simulink model "rst_auto_reg_Prototipo"  (R2015a)
settings: Solver=ode45  SolverMode=SingleTasking  StartTime=0.0  StopTime=50  RelTol=1e-3
values from neighbouring files (symbols this model uses):
  A = den    [cod_teste_RST_4.m]
  B = num    [cod_teste_RST_4.m]
  ep = 0.9    [cod_teste_RST_4.m]
  T = sum(Am)/sum(B)    [cod_teste_RST_4.m]
  Ts = 1    [cod_teste_RST_4.m]
undefined symbols (not defined in the file or in its folder): T_a
libraries: dspinverses x5
settings Model: CovMetricSettings=dwe  CovHtmlReporting=off  covSaveCumulativeToWorkspaceVar=off  CovSaveSingleToWorkspaceVar=off  CovExternalEMLEnable=on  Creator=Carlos Henrique  LastModifiedBy=controle
settings DataIOCC: LimitDataPoints=off  SaveFormat=Dataset
settings DebuggingCC: SFUnexpectedBacktrackingDiag=error  SFNoUnconditionalDefaultTransitionDiag=error
settings HardwareCC: ProdBitPerPointer=64  ProdLargestAtomicFloat=Float  ProdIntDivRoundTo=Zero  ProdEndianess=LittleEndian  ProdHWDeviceType=Specified
settings ModelReferenceCC: PropagateSignalLabelsOutOfModel=on
settings SFSimCC: SimUseLocalCustomCode=on
settings RTWCC: RTWUseLocalCustomCode=on
settings GRTTargetCC: TargetLangStandard=C99 (ISO)  GeneratePreprocessorConditionals=Use local settings

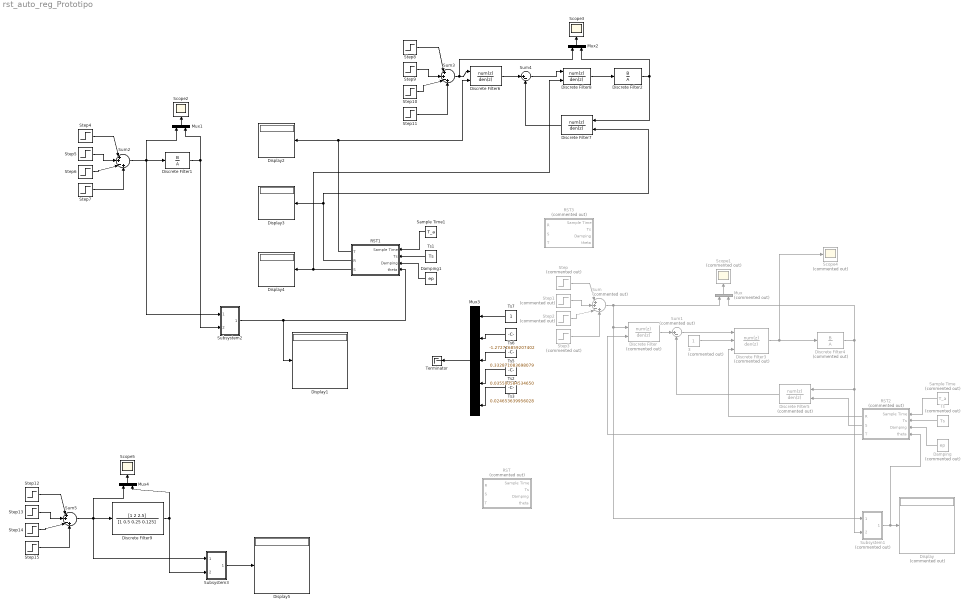
== system rst_auto_reg_Prototipo ==
  3 : Constant  Commented=on
  Damping : Constant  Commented=on  Value=ep
  Damping1 : Constant  Value=ep
  Discrete Filter : DiscreteFilter  Commented=on  NumeratorSource=Input port  Numerator=B  Denominator=1
      settings: InputPortMap=u0,p1
  Discrete Filter1 : DiscreteFilter  Numerator=B  Denominator=A  SampleTime=0.1
  Discrete Filter2 : DiscreteFilter  Numerator=B  Denominator=A  SampleTime=0.1
  Discrete Filter3 : DiscreteFilter  Commented=on  NumeratorSource=Input port  Numerator=T  DenominatorSource=Input port  Denominator=1  SampleTime=0.1  a0EqualsOne=on
      settings: InputPortMap=u0,p1,p3
  Discrete Filter4 : DiscreteFilter  Commented=on  Numerator=B  Denominator=A
  Discrete Filter5 : DiscreteFilter  Commented=on  NumeratorSource=Input port  Denominator=1
      settings: InputPortMap=u0,p1
  Discrete Filter6 : DiscreteFilter  NumeratorSource=Input port  Numerator=13.39  Denominator=1  SampleTime=0.1
      settings: InputPortMap=u0,p1
  Discrete Filter7 : DiscreteFilter  NumeratorSource=Input port  Numerator=[-0.6555 0.1406]  Denominator=1  SampleTime=0.1
      settings: InputPortMap=u0,p1
  Discrete Filter8 : DiscreteFilter  Numerator=1  DenominatorSource=Input port  Denominator=[0.634 -0.2621]  SampleTime=0.1  a0EqualsOne=on
      settings: InputPortMap=u0,p3
  Discrete Filter9 : DiscreteFilter  Numerator=[1 2 2.5]  Denominator=[1 0.5 0.25 0.125]  SampleTime=0.1
  Display : Display  Commented=on
  Display{1..5} (5 alike) : Display
  Mux : Mux  Commented=on  Inputs=2
  Mux1 : Mux  Inputs=2
  Mux2 : Mux  Inputs=2
  Mux3 : Mux  Inputs=5
  Mux4 : Mux  Inputs=2
  RST : Subsystem  Commented=on
  RST1 : Subsystem
  RST2 : Subsystem  Commented=on
  RST3 : Subsystem  Commented=on
  Sample Time : Constant  Commented=on  Value=T_a
  Sample Time1 : Constant  Value=T_a
  Scope1 : Scope  Commented=on
      settings: YMin=-0.73435  YMax=6.60919
  Scope2 : Scope
      settings: YMin=-0.73435  YMax=6.60919
  Scope3 : Scope
      settings: TimeRange=50  YMin=1.132890365448505  YMax=3.006644518272426  SaveName=ScopeData3
  Scope4 : Scope  Commented=on
      settings: YMin=-8.49296  YMax=18.39504  SaveName=ScopeData2
  Scope5 : Scope
      settings: YMin=-0.73435  YMax=6.60919  SaveName=ScopeData4
  Step : Step  Commented=on  Time=0  SampleTime=0
  Step1 : Step  Commented=on  Time=10  After=3  SampleTime=0
  Step10 : Step  Time=20  After=2  SampleTime=0
  Step11 : Step  Time=30  SampleTime=0
  Step12 : Step  Time=0  SampleTime=0
  Step13 : Step  Time=10  After=3  SampleTime=0
  Step14 : Step  Time=20  After=2  SampleTime=0
  Step15 : Step  Time=30  SampleTime=0
  Step2 : Step  Commented=on  Time=20  After=2  SampleTime=0
  Step3 : Step  Commented=on  Time=30  SampleTime=0
  Step4 : Step  Time=0  SampleTime=0
  Step5 : Step  Time=10  After=3  SampleTime=0
  Step6 : Step  Time=20  After=2  SampleTime=0
  Step7 : Step  Time=30  SampleTime=0
  Step8 : Step  Time=0  SampleTime=0
  Step9 : Step  Time=10  After=3  SampleTime=0
  Subsystem1 : Subsystem  Commented=on
  Subsystem2 : Subsystem
  Subsystem3 : Subsystem
  Sum : Sum  Commented=on  Inputs=|++-+
  Sum1 : Sum  Commented=on  Inputs=|+-
  Sum2 : Sum  Inputs=|++-+
  Sum3 : Sum  Inputs=|++-+
  Sum4 : Sum  Inputs=|+-
  Sum5 : Sum  Inputs=|++-+
  Terminator : Terminator
  Ts : Constant  Commented=on  Value=Ts
  Ts1 : Constant  Value=Ts
  Ts2 : Constant  Value=0.035500584534650  SampleTime=0.1
  Ts3 : Constant  Value=0.024653639956028  SampleTime=0.1
  Ts5 : Constant  Value=0.332871083698079  SampleTime=0.1
  Ts6 : Constant  Value=-1.272716859207402  SampleTime=0.1
  Ts7 : Constant  SampleTime=0.1
  wires:
  RST2/2(S) -> Discrete Filter5/2
  Mux/1 -> Scope1/1
  Ts/1 -> RST2/2(Ts)
  Step2/1 -> Sum/3
  Damping/1 -> RST2/3(Damping)
  RST2/1(R) -> Discrete Filter3/3
  Step1/1 -> Sum/2
  Discrete Filter3/1 -> Discrete Filter4/1, Scope4/1
  Sample Time/1 -> RST2/1(Sample Time)
  Sum/1 -> Subsystem1/1(In1), Discrete Filter/1, Mux/1
  Step3/1 -> Sum/4
  3/1 -> Discrete Filter3/2
  Sum1/1 -> Discrete Filter3/1
  Step/1 -> Sum/1
  RST2/3(T) -> Discrete Filter/2
  Discrete Filter/1 -> Sum1/1
  Discrete Filter5/1 -> Sum1/2
  Discrete Filter4/1 -> Subsystem1/2(In2), Discrete Filter5/1, Mux/2
  Sample Time1/1 -> RST1/1(Sample Time)
  Ts1/1 -> RST1/2(Ts)
  Damping1/1 -> RST1/3(Damping)
  Subsystem2/1(Out1) -> Display1/1, RST1/4(theta)
  Step5/1 -> Sum2/2
  Step7/1 -> Sum2/4
  Step6/1 -> Sum2/3
  Step4/1 -> Sum2/1
  Sum2/1 -> Subsystem2/1(In1), Mux1/1, Discrete Filter1/1
  Discrete Filter1/1 -> Subsystem2/2(In2), Mux1/2
  Mux1/1 -> Scope2/1
  RST1/1(T) -> Discrete Filter6/2, Display2/1
  Step8/1 -> Sum3/1
  Step10/1 -> Sum3/3
  Step11/1 -> Sum3/4
  Step9/1 -> Sum3/2
  Sum3/1 -> Mux2/1, Discrete Filter6/1
  Discrete Filter6/1 -> Sum4/1
  Discrete Filter7/1 -> Sum4/2
  Discrete Filter8/1 -> Discrete Filter2/1
  Discrete Filter2/1 -> Discrete Filter7/1, Mux2/2
  Subsystem1/1(Out1) -> RST2/4(theta), Display/1
  Ts7/1 -> Mux3/1
  Ts6/1 -> Mux3/2
  Ts5/1 -> Mux3/3
  Ts2/1 -> Mux3/4
  Ts3/1 -> Mux3/5
  Mux3/1 -> Terminator/1
  RST1/3(S) -> Discrete Filter8/2, Display4/1
  RST1/2(R) -> Discrete Filter7/2, Display3/1
  Sum4/1 -> Discrete Filter8/1
  Mux2/1 -> Scope3/1
  Step13/1 -> Sum5/2
  Step15/1 -> Sum5/4
  Step14/1 -> Sum5/3
  Step12/1 -> Sum5/1
  Sum5/1 -> Discrete Filter9/1, Mux4/1, Subsystem3/1(In1)
  Mux4/1 -> Scope5/1
  Subsystem3/1(Out1) -> Display5/1
  Discrete Filter9/1 -> Subsystem3/2(In2), Mux4/2

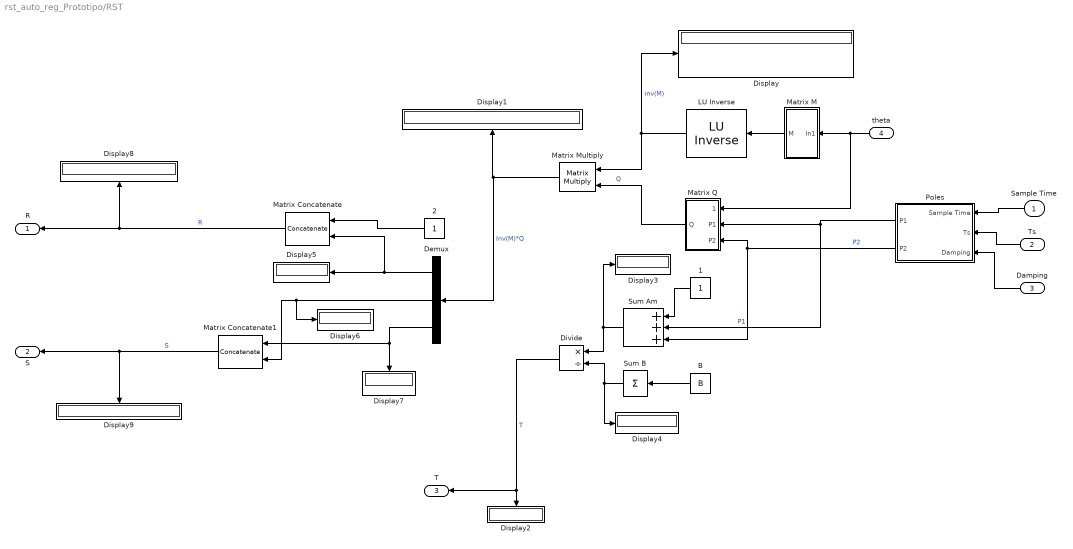
== system rst_auto_reg_Prototipo/RST ==
  Sample Time : Inport
  Ts : Inport  Port=2
  Damping : Inport  Port=3
  theta : Inport  Port=4
  " LU Inverse" : dspinverses/ LU Inverse
  1 : Constant
  2 : Constant
  B : Constant  Value=B
  Demux : Demux  Outputs=3
  Display{,1..9} (10 alike) : Display
  Divide : Product  Inputs=*/
  Matrix Concatenate : Concatenate  Mode=Multidimensional array  ConcatenateDimension=2
  Matrix Concatenate1 : Concatenate  Mode=Multidimensional array  ConcatenateDimension=2
  Matrix M : Subsystem
  Matrix Multiply : Product  Multiplication=Matrix(*)
  Matrix Q : Subsystem
  Poles : Subsystem
  Sum Am : Sum  Inputs=+++
  Sum B : Sum  Inputs=+
  R : Outport
  S : Outport  Port=2
  T : Outport  Port=3
  wires:
  Matrix Multiply/1 -> Demux/1, Display1/1  "Inv(M)*Q"
  Demux/1 -> Matrix Concatenate/2, Display5/1
  Sum B/1 -> Divide/2, Display4/1
  " LU Inverse"/1 -> Matrix Multiply/1, Display/1  "inv(M)"
  Matrix Concatenate/1 -> Display8/1, R/1  "R"
  B/1 -> Sum B/1
  Demux/2 -> Display6/1, Matrix Concatenate1/2
  Sum Am/1 -> Divide/1, Display3/1
  Matrix Concatenate1/1 -> S/1, Display9/1  "S"
  Poles/2(P2) -> Sum Am/3, Matrix Q/3(P2)  "P2"
  Divide/1 -> T/1, Display2/1  "T"
  Ts/1 -> Poles/2(Ts)
  Matrix Q/1(Q) -> Matrix Multiply/2  "Q"
  Damping/1 -> Poles/3(Damping)
  Sample Time/1 -> Poles/1(Sample Time)
  1/1 -> Sum Am/1
  Demux/3 -> Display7/1, Matrix Concatenate1/1
  2/1 -> Matrix Concatenate/1
  theta/1 -> Matrix Q/1(theta), Matrix M/1(In1)
  Matrix M/1(M) -> " LU Inverse"/1
  Poles/1(P1) -> Sum Am/2, Matrix Q/2(P1)  "P1"

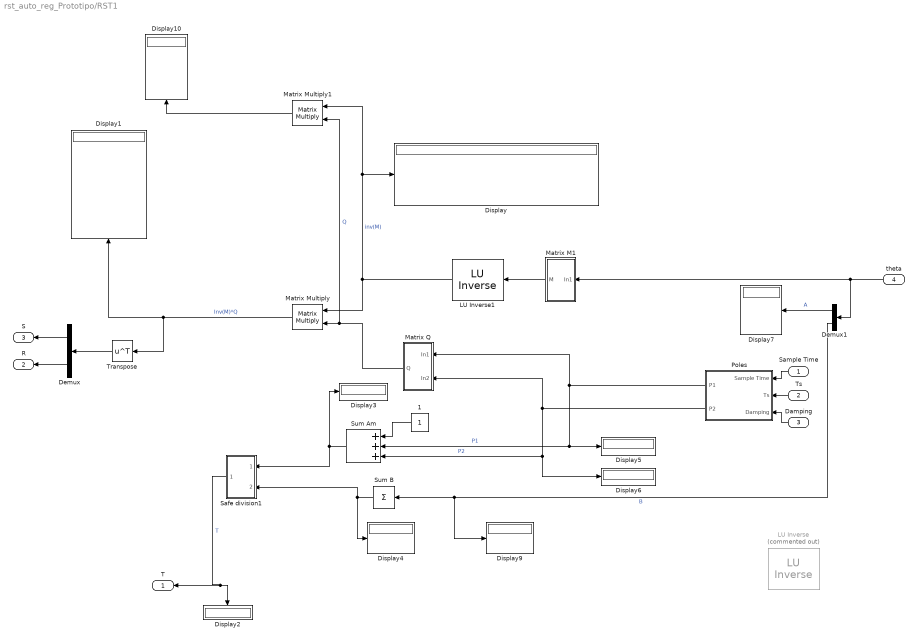
== system rst_auto_reg_Prototipo/RST1 ==
  Sample Time : Inport
  Ts : Inport  Port=2
  Damping : Inport  Port=3
  theta : Inport  Port=4
  " LU Inverse" : dspinverses/ LU Inverse  Commented=on
  " LU Inverse1" : dspinverses/ LU Inverse
  1 : Constant
  Demux : Demux  Outputs=2
  Demux1 : Demux  Outputs=2
  Display{,1..7,9..10} (10 alike) : Display
  Matrix M1 : Subsystem
  Matrix Multiply : Product  Multiplication=Matrix(*)
  Matrix Multiply1 : Product  Multiplication=Matrix(*)
  Matrix Q : Subsystem
  Poles : Subsystem
  Safe division1 : Subsystem
  Sum Am : Sum  Inputs=+++
  Sum B : Sum  Inputs=+
  Transpose : Math  Operator=transpose  SaturateOnIntegerOverflow=on
  T : Outport
  R : Outport  Port=2
  S : Outport  Port=3
  wires:
  Matrix Multiply/1 -> Transpose/1, Display1/1  "Inv(M)*Q"
  Sum B/1 -> Display4/1, Safe division1/2(In2)
  " LU Inverse1"/1 -> Matrix Multiply/1, Matrix Multiply1/1, Display/1  "inv(M)"
  Sum Am/1 -> Safe division1/1(In1), Display3/1
  Safe division1/1(Out1) -> Display2/1, T/1  "T"
  Ts/1 -> Poles/2(Ts)
  Matrix Q/1(Q) -> Matrix Multiply1/2, Matrix Multiply/2  "Q"
  Damping/1 -> Poles/3(Damping)
  Sample Time/1 -> Poles/1(Sample Time)
  1/1 -> Sum Am/1
  theta/1 -> Matrix M1/1(In1), Demux1/1
  Demux1/2 -> Display9/1, Sum B/1  "B"
  Demux1/1 -> Display7/1  "A"
  Poles/1(P1) -> Matrix Q/1(In1), Sum Am/2, Display5/1  "P1"
  Poles/2(P2) -> Display6/1, Sum Am/3, Matrix Q/2(In2)  "P2"
  Matrix M1/1(M) -> " LU Inverse1"/1
  Transpose/1 -> Demux/1
  Demux/1 -> S/1
  Demux/2 -> R/1
  Matrix Multiply1/1 -> Display10/1

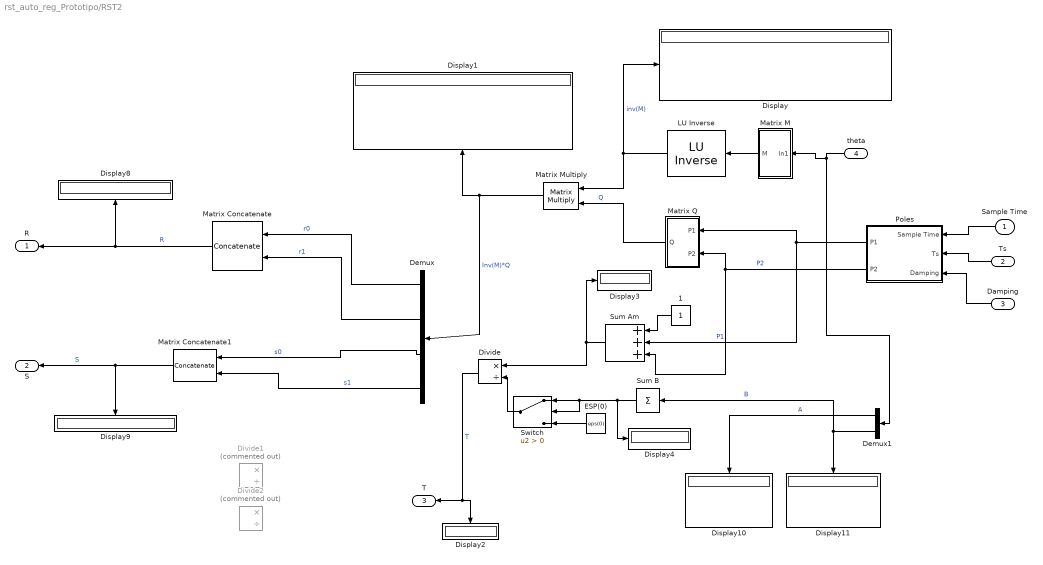
== system rst_auto_reg_Prototipo/RST2 ==
  Sample Time : Inport
  Ts : Inport  Port=2
  Damping : Inport  Port=3
  theta : Inport  Port=4
  " ESP(0)" : Constant  Value=eps(0)
  " LU Inverse" : dspinverses/ LU Inverse
  1 : Constant
  Demux : Demux
  Demux1 : Demux  Outputs=2
  Display{,1..4,8..11} (9 alike) : Display
  Divide : Product  Inputs=*/
  Divide1 : Product  Commented=on  Inputs=*/
  Divide2 : Product  Commented=on  Inputs=*/
  Matrix Concatenate : Concatenate  Mode=Multidimensional array  ConcatenateDimension=2
  Matrix Concatenate1 : Concatenate  Mode=Multidimensional array  ConcatenateDimension=2
  Matrix M : Subsystem
  Matrix Multiply : Product  Multiplication=Matrix(*)
  Matrix Q : Subsystem
  Poles : Subsystem
  Sum Am : Sum  Inputs=+++
  Sum B : Sum  Inputs=+
  Switch : Switch  Criteria=u2 > Threshold
  R : Outport
  S : Outport  Port=2
  T : Outport  Port=3
  wires:
  Demux/4 -> Matrix Concatenate1/2  "s1"
  Demux/3 -> Matrix Concatenate1/1  "s0"
  " ESP(0)"/1 -> Switch/3
  Switch/1 -> Divide/2
  Demux/2 -> Matrix Concatenate/2  "r1"
  Demux/1 -> Matrix Concatenate/1  "r0"
  Demux1/1 -> Display10/1  "A"
  Demux1/2 -> Display11/1, Sum B/1  "B"
  Poles/1(P1) -> Matrix Q/1(P1), Sum Am/2  "P1"
  Matrix M/1(M) -> " LU Inverse"/1
  theta/1 -> Matrix M/1(In1), Demux1/1
  1/1 -> Sum Am/1
  Sample Time/1 -> Poles/1(Sample Time)
  Damping/1 -> Poles/3(Damping)
  Matrix Q/1(Q) -> Matrix Multiply/2  "Q"
  Ts/1 -> Poles/2(Ts)
  Divide/1 -> T/1, Display2/1  "T"
  Poles/2(P2) -> Sum Am/3, Matrix Q/2(P2)  "P2"
  Matrix Concatenate1/1 -> Display9/1, S/1  "S"
  Sum Am/1 -> Display3/1, Divide/1
  Matrix Concatenate/1 -> R/1, Display8/1  "R"
  " LU Inverse"/1 -> Display/1, Matrix Multiply/1  "inv(M)"
  Sum B/1 -> Display4/1, Switch/1, Switch/2
  Matrix Multiply/1 -> Display1/1, Demux/1  "Inv(M)*Q"

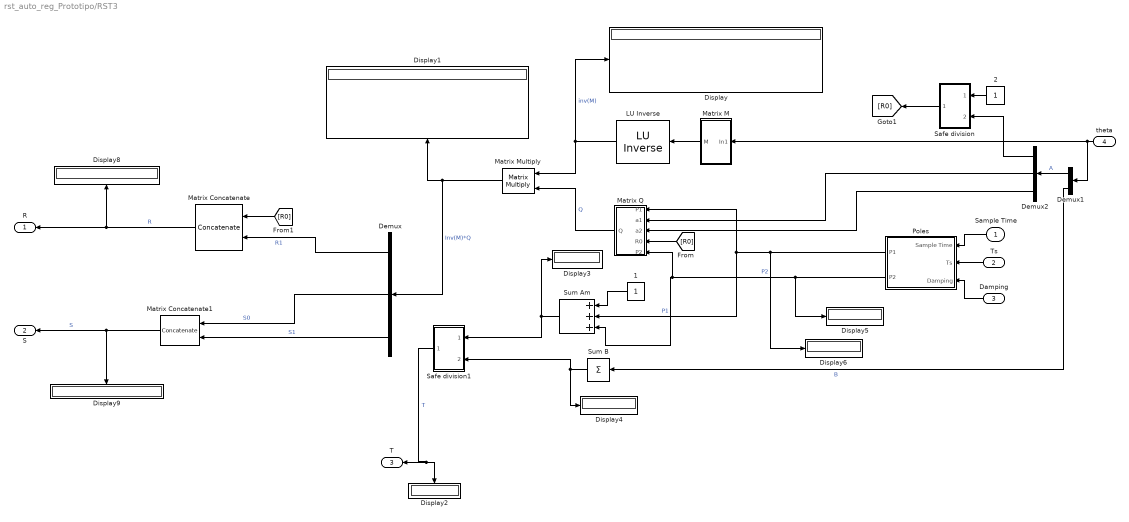
== system rst_auto_reg_Prototipo/RST3 ==
  Sample Time : Inport
  Ts : Inport  Port=2
  Damping : Inport  Port=3
  theta : Inport  Port=4
  " LU Inverse" : dspinverses/ LU Inverse
  1 : Constant
  2 : Constant
  Demux : Demux  Outputs=3
  Demux1 : Demux  Outputs=2
  Demux2 : Demux  Outputs=3
  Display{,1..6,8..9} (9 alike) : Display
  Matrix Concatenate : Concatenate  Mode=Multidimensional array  ConcatenateDimension=2
  Matrix Concatenate1 : Concatenate  Mode=Multidimensional array  ConcatenateDimension=2
  Matrix M : Subsystem
  Matrix Multiply : Product  Multiplication=Matrix(*)
  Matrix Q : Subsystem
  Poles : Subsystem
  Safe division : Subsystem
  Safe division1 : Subsystem
  Sum Am : Sum  Inputs=+++
  Sum B : Sum  Inputs=+
  R : Outport
  S : Outport  Port=2
  T : Outport  Port=3
  wires:
  Demux/1 -> Matrix Concatenate/2  "R1"
  Demux/3 -> Matrix Concatenate1/2  "S1"
  [R0] -> Matrix Concatenate/1
  [R0] -> Matrix Q/4(R0)
  Safe division/1(Out1) -> [R0]
  Demux/2 -> Matrix Concatenate1/1  "S0"
  Demux2/3 -> Matrix Q/3(a2)
  Demux2/2 -> Matrix Q/2(a1)
  2/1 -> Safe division/1(In1)
  Demux2/1 -> Safe division/2(In2)
  Demux1/1 -> Demux2/1  "A"
  Demux1/2 -> Sum B/1  "B"
  Poles/1(P1) -> Sum Am/2, Matrix Q/1(P1), Display6/1  "P1"
  Matrix M/1(M) -> " LU Inverse"/1
  theta/1 -> Demux1/1, Matrix M/1(In1)
  1/1 -> Sum Am/1
  Sample Time/1 -> Poles/1(Sample Time)
  Damping/1 -> Poles/3(Damping)
  Matrix Q/1(Q) -> Matrix Multiply/2  "Q"
  Ts/1 -> Poles/2(Ts)
  Safe division1/1(Out1) -> T/1, Display2/1  "T"
  Poles/2(P2) -> Sum Am/3, Matrix Q/5(P2), Display5/1  "P2"
  Matrix Concatenate1/1 -> S/1, Display9/1  "S"
  Sum Am/1 -> Display3/1, Safe division1/1(In1)
  Matrix Concatenate/1 -> R/1, Display8/1  "R"
  " LU Inverse"/1 -> Display/1, Matrix Multiply/1  "inv(M)"
  Sum B/1 -> Safe division1/2(In2), Display4/1
  Matrix Multiply/1 -> Display1/1, Demux/1  "Inv(M)*Q"

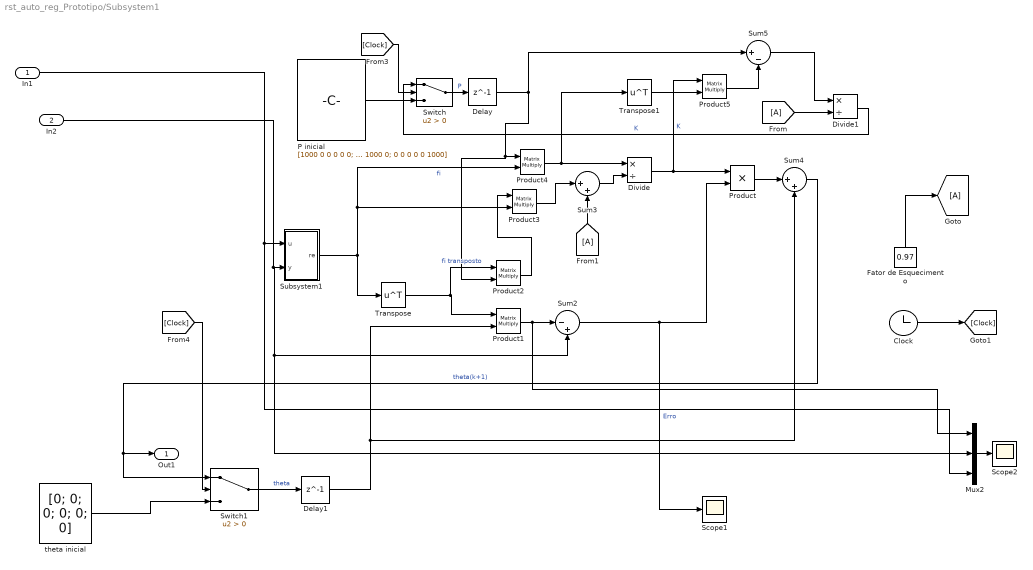
== system rst_auto_reg_Prototipo/Subsystem1 ==
  In1 : Inport
  In2 : Inport  Port=2
  Clock : Clock
  Delay : Delay  DelayLength=1  InitialCondition=0  SampleTime=0.1
  Delay1 : Delay  DelayLength=1  InitialCondition=0  SampleTime=0.1
  Divide : Product  Inputs=*/
  Divide1 : Product  Inputs=*/
  "Fator de Esquecimento " : Constant  Value=0.97
  Mux2 : Mux  Inputs=3
  P inicial : Constant  Value=[1000 0 0 0 0 0; 0 1000 0 0 0 0; 0 0 1000 0 0 0; 0 0 0 1000 0 0; 0 0 0 0 1000 0; 0 0 0 0 0 1000]
  Product : Product
  Product{1..5} (5 alike) : Product  Multiplication=Matrix(*)
  Scope1 : Scope
      settings: YMin=-0.1368  YMax=1.23123
  Scope2 : Scope
      settings: YMin=-0.50752  YMax=4.51143
  Subsystem1 : Subsystem
  Sum2 : Sum  Inputs=|-+
  Sum3 : Sum  Inputs=|++
  Sum4 : Sum  Inputs=|++
  Sum5 : Sum  Inputs=|+-
  Switch : Switch  Criteria=u2 > Threshold
  Switch1 : Switch  Criteria=u2 > Threshold
  Transpose : Math  Operator=transpose  SaturateOnIntegerOverflow=on
  Transpose1 : Math  Operator=transpose  SaturateOnIntegerOverflow=on
  "theta inicial " : Constant  Value=[0; 0; 0; 0; 0; 0]
  Out1 : Outport
  wires:
  Subsystem1/1(re) -> Transpose/1, Product4/2, Product3/2  "fi"
  Product/1 -> Sum4/1
  In2/1 -> Mux2/2, Sum2/2, Subsystem1/2(y)
  "Fator de Esquecimento "/1 -> [A]
  Transpose/1 -> Product2/1, Product1/1  "fi transposto"
  Sum3/1 -> Divide/2
  Product3/1 -> Sum3/1
  Switch/1 -> Delay/1  "P"
  Product4/1 -> Transpose1/1, Divide/1
  Delay/1 -> Product2/2, Product4/1, Sum5/1
  Divide/1 -> Product5/1, Product/1  "K"
  Transpose1/1 -> Product5/2
  Sum5/1 -> Divide1/1
  Sum2/1 -> Scope1/1, Product/2  "Erro"
  Delay1/1 -> Sum4/2, Product1/2
  Divide1/1 -> Switch/1  "K"
  "theta inicial "/1 -> Switch1/3
  [A] -> Divide1/2
  Product2/1 -> Product3/1
  Clock/1 -> [Clock]
  Product1/1 -> Mux2/1, Sum2/1
  Product5/1 -> Sum5/2
  P inicial/1 -> Switch/3
  Sum4/1 -> Out1/1, Switch1/1  "theta(k+1)"
  [A] -> Sum3/2
  In1/1 -> Mux2/3, Subsystem1/1(u)
  [Clock] -> Switch/2
  Switch1/1 -> Delay1/1  "theta"
  Mux2/1 -> Scope2/1
  [Clock] -> Switch1/2

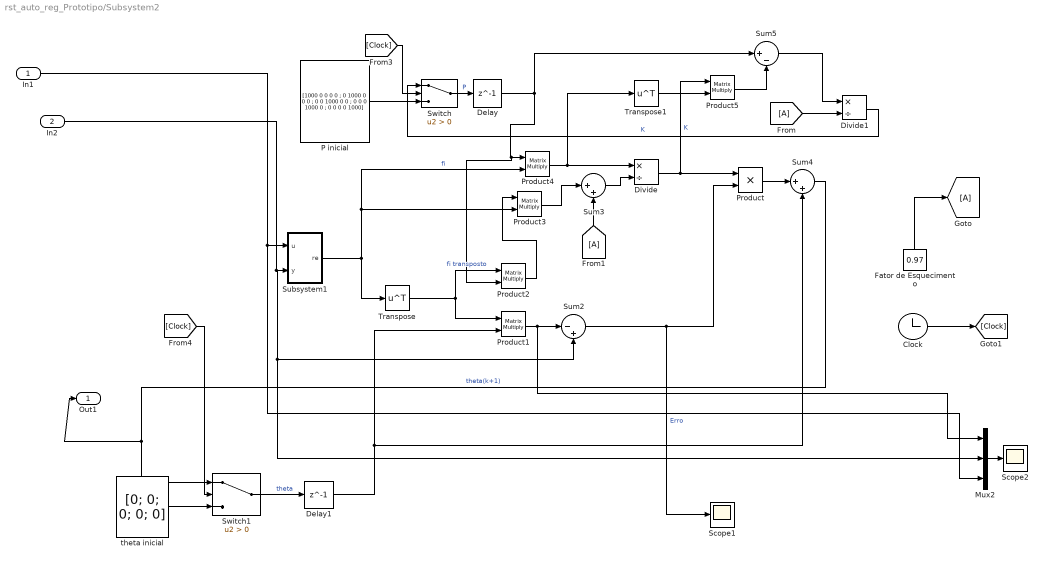
== system rst_auto_reg_Prototipo/Subsystem2 ==
  In1 : Inport
  In2 : Inport  Port=2
  Clock : Clock
  Delay : Delay  DelayLength=1  InitialCondition=0  SampleTime=0.1
  Delay1 : Delay  DelayLength=1  InitialCondition=0  SampleTime=0.1
  Divide : Product  Inputs=*/
  Divide1 : Product  Inputs=*/
  "Fator de Esquecimento " : Constant  Value=0.97
  Mux2 : Mux  Inputs=3
  P inicial : Constant  Value=[1000 0 0 0 0 ; 0 1000 0 0 0 ; 0 0 1000 0 0 ; 0 0 0 1000 0 ; 0 0 0 0 1000]  SampleTime=0.1
  Product : Product
  Product{1..5} (5 alike) : Product  Multiplication=Matrix(*)
  Scope1 : Scope
      settings: YMin=-0.1368  YMax=1.23123
  Scope2 : Scope
      settings: YMin=-0.50752  YMax=4.51143
  Subsystem1 : Subsystem
  Sum2 : Sum  Inputs=|-+
  Sum3 : Sum  Inputs=|++
  Sum4 : Sum  Inputs=|++
  Sum5 : Sum  Inputs=|+-
  Switch : Switch  Criteria=u2 > Threshold
  Switch1 : Switch  Criteria=u2 > Threshold
  Transpose : Math  Operator=transpose  SaturateOnIntegerOverflow=on
  Transpose1 : Math  Operator=transpose  SaturateOnIntegerOverflow=on
  "theta inicial " : Constant  Value=[0; 0; 0; 0; 0]  SampleTime=0.1
  Out1 : Outport
  wires:
  Subsystem1/1(re) -> Transpose/1, Product4/2, Product3/2  "fi"
  Product/1 -> Sum4/1
  In2/1 -> Mux2/2, Sum2/2, Subsystem1/2(y)
  "Fator de Esquecimento "/1 -> [A]
  Transpose/1 -> Product2/1, Product1/1  "fi transposto"
  Sum3/1 -> Divide/2
  Product3/1 -> Sum3/1
  Switch/1 -> Delay/1  "P"
  Product4/1 -> Transpose1/1, Divide/1
  Delay/1 -> Product2/2, Product4/1, Sum5/1
  Divide/1 -> Product5/1, Product/1  "K"
  Transpose1/1 -> Product5/2
  Sum5/1 -> Divide1/1
  Sum2/1 -> Scope1/1, Product/2  "Erro"
  Delay1/1 -> Sum4/2, Product1/2
  Divide1/1 -> Switch/1  "K"
  "theta inicial "/1 -> Switch1/3
  [A] -> Divide1/2
  Product2/1 -> Product3/1
  Clock/1 -> [Clock]
  Product1/1 -> Mux2/1, Sum2/1
  Product5/1 -> Sum5/2
  P inicial/1 -> Switch/3
  Sum4/1 -> Out1/1, Switch1/1  "theta(k+1)"
  [A] -> Sum3/2
  In1/1 -> Mux2/3, Subsystem1/1(u)
  [Clock] -> Switch/2
  Switch1/1 -> Delay1/1  "theta"
  Mux2/1 -> Scope2/1
  [Clock] -> Switch1/2

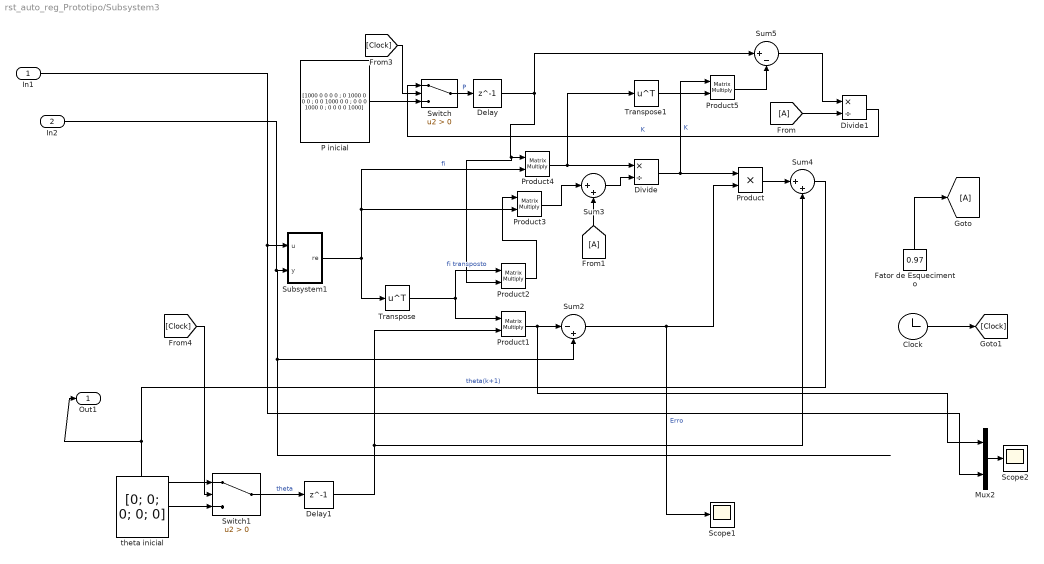
== system rst_auto_reg_Prototipo/Subsystem3 ==
  In1 : Inport
  In2 : Inport  Port=2
  Clock : Clock
  Delay : Delay  DelayLength=1  InitialCondition=0  SampleTime=0.1
  Delay1 : Delay  DelayLength=1  InitialCondition=0  SampleTime=0.1
  Divide : Product  Inputs=*/
  Divide1 : Product  Inputs=*/
  "Fator de Esquecimento " : Constant  Value=0.97
  Mux2 : Mux  Inputs=2
  P inicial : Constant  Value=[1000 0 0 0 0 ; 0 1000 0 0 0 ; 0 0 1000 0 0 ; 0 0 0 1000 0 ; 0 0 0 0 1000]  SampleTime=0.1
  Product : Product
  Product{1..5} (5 alike) : Product  Multiplication=Matrix(*)
  Scope1 : Scope
      settings: YMin=-0.1368  YMax=1.23123
  Scope2 : Scope
      settings: TimeRange=20  YMin=0.1724517906336078  YMax=1.772451790633608
  Subsystem1 : Subsystem
  Sum2 : Sum  Inputs=|-+
  Sum3 : Sum  Inputs=|++
  Sum4 : Sum  Inputs=|++
  Sum5 : Sum  Inputs=|+-
  Switch : Switch  Criteria=u2 > Threshold
  Switch1 : Switch  Criteria=u2 > Threshold
  Transpose : Math  Operator=transpose  SaturateOnIntegerOverflow=on
  Transpose1 : Math  Operator=transpose  SaturateOnIntegerOverflow=on
  "theta inicial " : Constant  Value=[0; 0; 0; 0; 0]  SampleTime=0.1
  Out1 : Outport
  wires:
  Subsystem1/1(re) -> Transpose/1, Product4/2, Product3/2  "fi"
  Product/1 -> Sum4/1
  In2/1 -> Sum2/2, Subsystem1/2(y)
  "Fator de Esquecimento "/1 -> [A]
  Transpose/1 -> Product2/1, Product1/1  "fi transposto"
  Sum3/1 -> Divide/2
  Product3/1 -> Sum3/1
  Switch/1 -> Delay/1  "P"
  Product4/1 -> Transpose1/1, Divide/1
  Delay/1 -> Product2/2, Product4/1, Sum5/1
  Divide/1 -> Product5/1, Product/1  "K"
  Transpose1/1 -> Product5/2
  Sum5/1 -> Divide1/1
  Sum2/1 -> Scope1/1, Product/2  "Erro"
  Delay1/1 -> Sum4/2, Product1/2
  Divide1/1 -> Switch/1  "K"
  "theta inicial "/1 -> Switch1/3
  [A] -> Divide1/2
  Product2/1 -> Product3/1
  Clock/1 -> [Clock]
  Product1/1 -> Mux2/1, Sum2/1
  Product5/1 -> Sum5/2
  P inicial/1 -> Switch/3
  Sum4/1 -> Out1/1, Switch1/1  "theta(k+1)"
  [A] -> Sum3/2
  In1/1 -> Mux2/2, Subsystem1/1(u)
  [Clock] -> Switch/2
  Switch1/1 -> Delay1/1  "theta"
  Mux2/1 -> Scope2/1
  [Clock] -> Switch1/2

== system rst_auto_reg_Prototipo/RST/Matrix M ==
  In1 : Inport
  " " : Constant  Value=0
  1 : Constant
  Demux : Demux  Outputs=6
  Display : Display
  Matrix Concatenate{,1..5} (6 alike) : Concatenate  Mode=Multidimensional array  ConcatenateDimension=2
  Matrix Concatenate6 : Concatenate  Mode=Multidimensional array
  Matrix Concatenate7 : Concatenate  Mode=Multidimensional array
  Terminator : Terminator
  Terminator1 : Terminator
  M : Outport
  wires:
  Demux/6 -> Matrix Concatenate4/2, Matrix Concatenate3/2  "b3"
  Demux/4 -> Terminator/1
  Demux/3 -> Matrix Concatenate4/1  "a3"
  In1/1 -> Demux/1
  Demux/5 -> Matrix Concatenate2/2, Matrix Concatenate1/2  "b2"
  Demux/2 -> Matrix Concatenate2/1  "a2"
  " "/1 -> Matrix Concatenate/2, Matrix Concatenate5/2
  Demux/1 -> Terminator1/1  "a1"
  Matrix Concatenate4/1 -> Matrix Concatenate5/1
  1/1 -> Matrix Concatenate/1
  Matrix Concatenate5/1 -> Matrix Concatenate7/2
  Matrix Concatenate2/1 -> Matrix Concatenate3/1
  Matrix Concatenate/1 -> Matrix Concatenate1/1
  Matrix Concatenate6/1 -> Matrix Concatenate7/1
  Matrix Concatenate3/1 -> Matrix Concatenate6/2
  Matrix Concatenate7/1 -> M/1, Display/1
  Matrix Concatenate1/1 -> Matrix Concatenate6/1

== system rst_auto_reg_Prototipo/RST/Matrix Q ==
  theta : Inport
  P1 : Inport  Port=2
  P2 : Inport  Port=3
  0 : Constant  Value=0
  Demux : Demux  Outputs=6
  Display : Display
  Matrix Concatenate : Concatenate  Mode=Multidimensional array
  Matrix Concatenate1 : Concatenate  Mode=Multidimensional array
  Subtract : Sum  Inputs=+-
  Subtract1 : Sum  Inputs=+-
  Terminator{,1..3} (4 alike) : Terminator
  Q : Outport
  wires:
  Subtract1/1 -> Matrix Concatenate/2
  Matrix Concatenate/1 -> Matrix Concatenate1/1
  Subtract/1 -> Matrix Concatenate/1
  Matrix Concatenate1/1 -> Q/1, Display/1
  P1/1 -> Subtract/1
  0/1 -> Matrix Concatenate1/2
  P2/1 -> Subtract1/1
  theta/1 -> Demux/1
  Demux/6 -> Terminator1/1  "b3"
  Demux/5 -> Terminator/1  "b2"
  Demux/4 -> Terminator2/1
  Demux/1 -> Terminator3/1  "a1"
  Demux/2 -> Subtract/2  "a2"
  Demux/3 -> Subtract1/2  "a3"

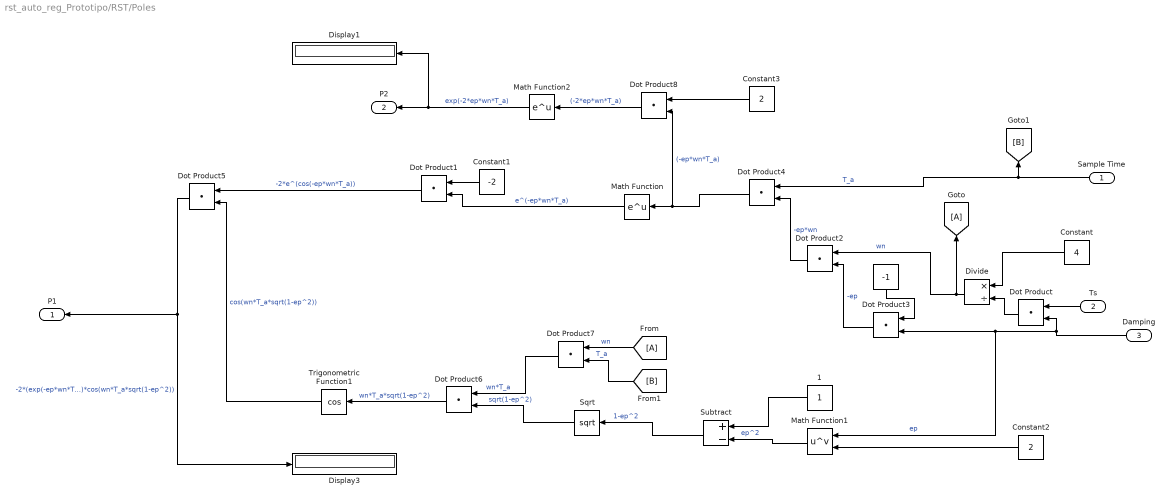
== system rst_auto_reg_Prototipo/RST/Poles ==
  Sample Time : Inport
  Ts : Inport  Port=2
  Damping : Inport  Port=3
  " " : Constant  Value=-1
  1 : Constant
  Constant : Constant  Value=4
  Constant1 : Constant  Value=-2
  Constant2 : Constant  Value=2
  Constant3 : Constant  Value=2
  Display1 : Display
  Display3 : Display
  Divide : Product  Inputs=*/
  Dot Product{,1..8} (9 alike) : DotProduct  InputSameDT=on  OutDataTypeStr=Inherit: Inherit via internal rule
  Math Function : Math  SaturateOnIntegerOverflow=on
  Math Function1 : Math  Operator=pow  SaturateOnIntegerOverflow=on
  Math Function2 : Math  SaturateOnIntegerOverflow=on
  Sqrt : Sqrt  SaturateOnIntegerOverflow=on
  Subtract : Sum  Inputs=+-
  Trigonometric Function1 : Trigonometry  Operator=cos
  P1 : Outport
  P2 : Outport  Port=2
  wires:
  Math Function/1 -> Dot Product1/2  "e^(-ep*wn*T_a)"
  Divide/1 -> [A], Dot Product2/1  "wn"
  [A] -> Dot Product7/1  "wn"
  " "/1 -> Dot Product3/1
  Dot Product5/1 -> P1/1, Display3/1  "-2*(exp(-ep*wn*T_a))*cos(wn*T_a*sqrt(1-ep^2))"
  Trigonometric Function1/1 -> Dot Product5/2  "cos(wn*T_a*sqrt(1-ep^2))"
  Ts/1 -> Dot Product/1
  Dot Product/1 -> Divide/2
  Dot Product3/1 -> Dot Product2/2  "-ep"
  Damping/1 -> Math Function1/1, Dot Product3/2, Dot Product/2  "ep"
  Constant/1 -> Divide/1
  Dot Product7/1 -> Dot Product6/1  "wn*T_a"
  Sample Time/1 -> Dot Product4/1, [B]  "T_a"
  Math Function1/1 -> Subtract/2  "ep^2"
  Dot Product1/1 -> Dot Product5/1  "-2*e^(cos(-ep*wn*T_a))"
  Constant2/1 -> Math Function1/2
  1/1 -> Subtract/1
  Constant1/1 -> Dot Product1/1
  Dot Product2/1 -> Dot Product4/2  "-ep*wn"
  [B] -> Dot Product7/2  "T_a"
  Dot Product6/1 -> Trigonometric Function1/1  "wn*T_a*sqrt(1-ep^2)"
  Dot Product4/1 -> Dot Product8/2, Math Function/1  "(-ep*wn*T_a)"
  Sqrt/1 -> Dot Product6/2  "sqrt(1-ep^2)"
  Subtract/1 -> Sqrt/1  "1-ep^2"
  Constant3/1 -> Dot Product8/1
  Dot Product8/1 -> Math Function2/1  "(-2*ep*wn*T_a)"
  Math Function2/1 -> Display1/1, P2/1  "exp(-2*ep*wn*T_a)"

== system rst_auto_reg_Prototipo/RST1/Matrix M1 ==
  In1 : Inport
  " " : Constant  Value=0
  Demux : Demux  Outputs=5
  Display : Display
  Matrix Concatenate{1..4} (4 alike) : Concatenate  NumInputs=4  Mode=Multidimensional array  ConcatenateDimension=2
  Matrix Concatenate6 : Concatenate  NumInputs=4  Mode=Multidimensional array
  M : Outport
  wires:
  Matrix Concatenate1/1 -> Matrix Concatenate6/1
  Demux/1 -> Matrix Concatenate2/2, Matrix Concatenate1/1  "a0"
  Matrix Concatenate6/1 -> M/1, Display/1
  In1/1 -> Demux/1
  Matrix Concatenate3/1 -> Matrix Concatenate6/3
  Matrix Concatenate4/1 -> Matrix Concatenate6/4
  Matrix Concatenate2/1 -> Matrix Concatenate6/2
  " "/1 -> Matrix Concatenate4/3, Matrix Concatenate4/1, Matrix Concatenate2/4, Matrix Concatenate1/4, Matrix Concatenate1/2, Matrix Concatenate1/3
  Demux/2 -> Matrix Concatenate3/2, Matrix Concatenate2/1  "a1"
  Demux/3 -> Matrix Concatenate4/2, Matrix Concatenate3/1  "a2"
  Demux/4 -> Matrix Concatenate3/4  "b1"
  Demux/5 -> Matrix Concatenate4/4, Matrix Concatenate2/3, Matrix Concatenate3/3  "b2"

== system rst_auto_reg_Prototipo/RST1/Matrix Q ==
  In1 : Inport
  In2 : Inport  Port=2
  0 : Constant  Value=0
  1 : Constant
  Display : Display
  Matrix Concatenate : Concatenate  NumInputs=4  Mode=Multidimensional array
  Q : Outport
  wires:
  Matrix Concatenate/1 -> Q/1, Display/1
  0/1 -> Matrix Concatenate/4
  1/1 -> Matrix Concatenate/1
  In1/1 -> Matrix Concatenate/2
  In2/1 -> Matrix Concatenate/3

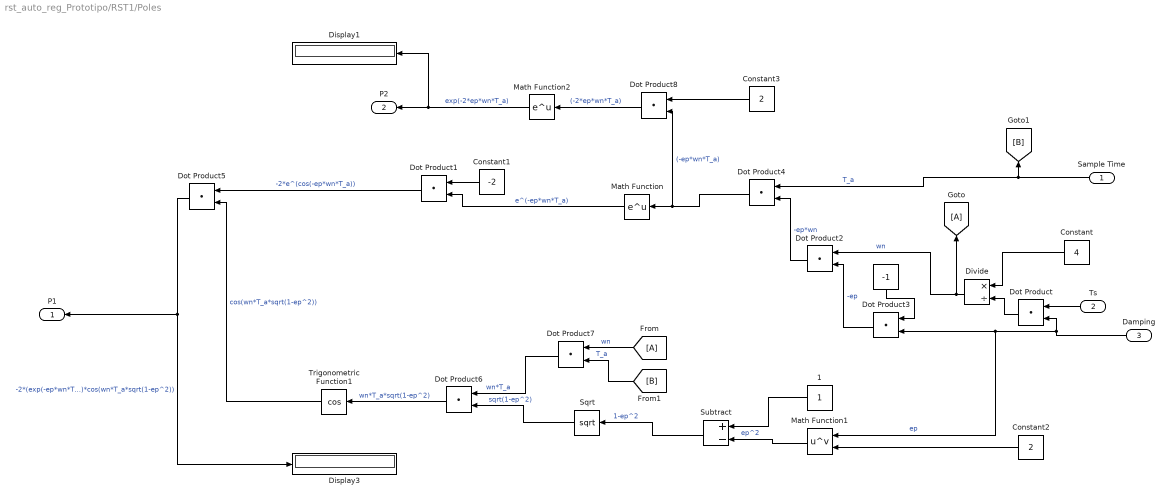
== system rst_auto_reg_Prototipo/RST1/Poles ==
  Sample Time : Inport
  Ts : Inport  Port=2
  Damping : Inport  Port=3
  " " : Constant  Value=-1
  1 : Constant
  Constant : Constant  Value=4
  Constant1 : Constant  Value=-2
  Constant2 : Constant  Value=2
  Constant3 : Constant  Value=2
  Display1 : Display
  Display3 : Display
  Divide : Product  Inputs=*/
  Dot Product{,1..8} (9 alike) : DotProduct  InputSameDT=on  OutDataTypeStr=Inherit: Inherit via internal rule
  Math Function : Math  SaturateOnIntegerOverflow=on
  Math Function1 : Math  Operator=pow  SaturateOnIntegerOverflow=on
  Math Function2 : Math  SaturateOnIntegerOverflow=on
  Sqrt : Sqrt  SaturateOnIntegerOverflow=on
  Subtract : Sum  Inputs=+-
  Trigonometric Function1 : Trigonometry  Operator=cos
  P1 : Outport
  P2 : Outport  Port=2
  wires:
  Math Function/1 -> Dot Product1/2  "e^(-ep*wn*T_a)"
  Divide/1 -> [A], Dot Product2/1  "wn"
  [A] -> Dot Product7/1  "wn"
  " "/1 -> Dot Product3/1
  Dot Product5/1 -> P1/1, Display3/1  "-2*(exp(-ep*wn*T_a))*cos(wn*T_a*sqrt(1-ep^2))"
  Trigonometric Function1/1 -> Dot Product5/2  "cos(wn*T_a*sqrt(1-ep^2))"
  Ts/1 -> Dot Product/1
  Dot Product/1 -> Divide/2
  Dot Product3/1 -> Dot Product2/2  "-ep"
  Damping/1 -> Math Function1/1, Dot Product3/2, Dot Product/2  "ep"
  Constant/1 -> Divide/1
  Dot Product7/1 -> Dot Product6/1  "wn*T_a"
  Sample Time/1 -> Dot Product4/1, [B]  "T_a"
  Math Function1/1 -> Subtract/2  "ep^2"
  Dot Product1/1 -> Dot Product5/1  "-2*e^(cos(-ep*wn*T_a))"
  Constant2/1 -> Math Function1/2
  1/1 -> Subtract/1
  Constant1/1 -> Dot Product1/1
  Dot Product2/1 -> Dot Product4/2  "-ep*wn"
  [B] -> Dot Product7/2  "T_a"
  Dot Product6/1 -> Trigonometric Function1/1  "wn*T_a*sqrt(1-ep^2)"
  Dot Product4/1 -> Dot Product8/2, Math Function/1  "(-ep*wn*T_a)"
  Sqrt/1 -> Dot Product6/2  "sqrt(1-ep^2)"
  Subtract/1 -> Sqrt/1  "1-ep^2"
  Constant3/1 -> Dot Product8/1
  Dot Product8/1 -> Math Function2/1  "(-2*ep*wn*T_a)"
  Math Function2/1 -> Display1/1, P2/1  "exp(-2*ep*wn*T_a)"

== system rst_auto_reg_Prototipo/RST1/Safe division1 ==
  In1 : Inport
  In2 : Inport  Port=2
  " ESP(0)1" : Constant  Value=eps(0)
  Divide3 : Product  Inputs=*/
  Switch1 : Switch  Criteria=u2 > Threshold
  Out1 : Outport
  wires:
  Divide3/1 -> Out1/1
  In1/1 -> Divide3/1
  In2/1 -> Switch1/2, Switch1/1
  " ESP(0)1"/1 -> Switch1/3
  Switch1/1 -> Divide3/2

== system rst_auto_reg_Prototipo/RST2/Matrix M ==
  In1 : Inport
  " " : Constant  Value=0
  Demux : Demux  Outputs=6
  Display : Display
  Matrix Concatenate{,1..3} (4 alike) : Concatenate  NumInputs=4  Mode=Multidimensional array  ConcatenateDimension=2
  Matrix Concatenate6 : Concatenate  NumInputs=4  Mode=Multidimensional array
  M : Outport
  wires:
  Matrix Concatenate3/1 -> Matrix Concatenate6/4
  Matrix Concatenate1/1 -> Matrix Concatenate6/3
  Matrix Concatenate2/1 -> Matrix Concatenate6/2
  Matrix Concatenate/1 -> Matrix Concatenate6/1
  Matrix Concatenate6/1 -> Display/1, M/1
  Demux/6 -> Matrix Concatenate1/3, Matrix Concatenate3/4  "b2"
  Demux/5 -> Matrix Concatenate1/4, Matrix Concatenate2/3  "b1"
  Demux/3 -> Matrix Concatenate1/1, Matrix Concatenate3/2  "a2"
  Demux/2 -> Matrix Concatenate1/2, Matrix Concatenate2/1  "a1"
  Demux/4 -> Matrix Concatenate2/4, Matrix Concatenate/3  "b0"
  " "/1 -> Matrix Concatenate/2, Matrix Concatenate/4, Matrix Concatenate3/1, Matrix Concatenate3/3
  Demux/1 -> Matrix Concatenate2/2, Matrix Concatenate/1  "a0"
  In1/1 -> Demux/1

== system rst_auto_reg_Prototipo/RST2/Matrix Q ==
  P1 : Inport
  P2 : Inport  Port=2
  0 : Constant  Value=0
  1 : Constant
  Display : Display
  Matrix Concatenate : Concatenate  NumInputs=4  Mode=Multidimensional array
  Q : Outport
  wires:
  0/1 -> Matrix Concatenate/4
  P2/1 -> Matrix Concatenate/3
  P1/1 -> Matrix Concatenate/2
  1/1 -> Matrix Concatenate/1
  Matrix Concatenate/1 -> Display/1, Q/1

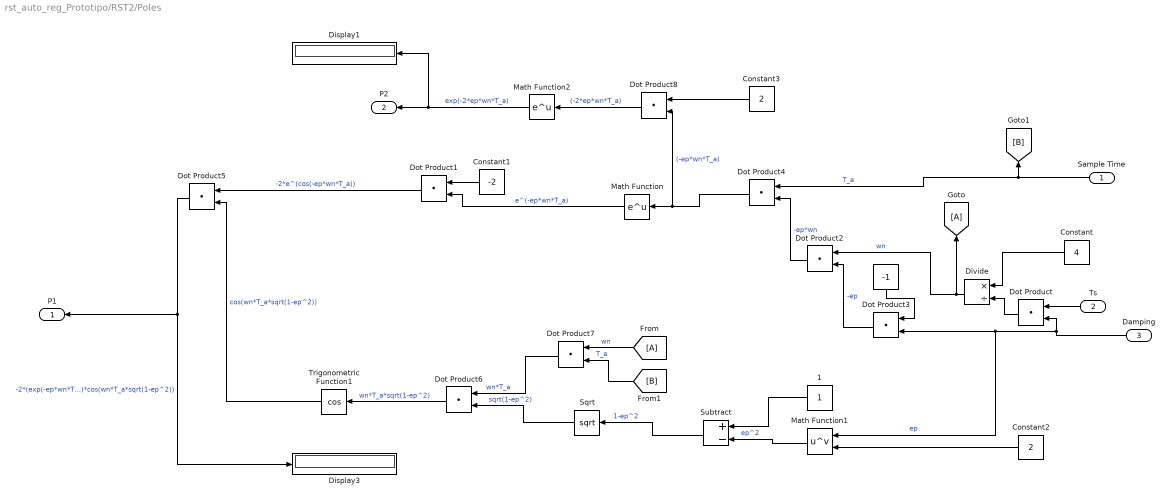
== system rst_auto_reg_Prototipo/RST2/Poles ==
  Sample Time : Inport
  Ts : Inport  Port=2
  Damping : Inport  Port=3
  " " : Constant  Value=-1
  1 : Constant
  Constant : Constant  Value=4
  Constant1 : Constant  Value=-2
  Constant2 : Constant  Value=2
  Constant3 : Constant  Value=2
  Display1 : Display
  Display3 : Display
  Divide : Product  Inputs=*/
  Dot Product{,1..8} (9 alike) : DotProduct  InputSameDT=on  OutDataTypeStr=Inherit: Inherit via internal rule
  Math Function : Math  SaturateOnIntegerOverflow=on
  Math Function1 : Math  Operator=pow  SaturateOnIntegerOverflow=on
  Math Function2 : Math  SaturateOnIntegerOverflow=on
  Sqrt : Sqrt  SaturateOnIntegerOverflow=on
  Subtract : Sum  Inputs=+-
  Trigonometric Function1 : Trigonometry  Operator=cos
  P1 : Outport
  P2 : Outport  Port=2
  wires:
  Math Function2/1 -> P2/1, Display1/1  "exp(-2*ep*wn*T_a)"
  Dot Product8/1 -> Math Function2/1  "(-2*ep*wn*T_a)"
  Constant3/1 -> Dot Product8/1
  Subtract/1 -> Sqrt/1  "1-ep^2"
  Sqrt/1 -> Dot Product6/2  "sqrt(1-ep^2)"
  Dot Product4/1 -> Math Function/1, Dot Product8/2  "(-ep*wn*T_a)"
  Dot Product6/1 -> Trigonometric Function1/1  "wn*T_a*sqrt(1-ep^2)"
  [B] -> Dot Product7/2  "T_a"
  Dot Product2/1 -> Dot Product4/2  "-ep*wn"
  Constant1/1 -> Dot Product1/1
  1/1 -> Subtract/1
  Constant2/1 -> Math Function1/2
  Dot Product1/1 -> Dot Product5/1  "-2*e^(cos(-ep*wn*T_a))"
  Math Function1/1 -> Subtract/2  "ep^2"
  Sample Time/1 -> [B], Dot Product4/1  "T_a"
  Dot Product7/1 -> Dot Product6/1  "wn*T_a"
  Constant/1 -> Divide/1
  Damping/1 -> Dot Product/2, Dot Product3/2, Math Function1/1  "ep"
  Dot Product3/1 -> Dot Product2/2  "-ep"
  Dot Product/1 -> Divide/2
  Ts/1 -> Dot Product/1
  Trigonometric Function1/1 -> Dot Product5/2  "cos(wn*T_a*sqrt(1-ep^2))"
  Dot Product5/1 -> Display3/1, P1/1  "-2*(exp(-ep*wn*T_a))*cos(wn*T_a*sqrt(1-ep^2))"
  " "/1 -> Dot Product3/1
  [A] -> Dot Product7/1  "wn"
  Divide/1 -> Dot Product2/1, [A]  "wn"
  Math Function/1 -> Dot Product1/2  "e^(-ep*wn*T_a)"

== system rst_auto_reg_Prototipo/RST3/Matrix M ==
  In1 : Inport
  " " : Constant  Value=0
  Demux : Demux  Outputs=5
  Display : Display
  Matrix Concatenate1 : Concatenate  NumInputs=3  Mode=Multidimensional array  ConcatenateDimension=2
  Matrix Concatenate2 : Concatenate  NumInputs=3  Mode=Multidimensional array  ConcatenateDimension=2
  Matrix Concatenate3 : Concatenate  NumInputs=3  Mode=Multidimensional array  ConcatenateDimension=2
  Matrix Concatenate6 : Concatenate  NumInputs=3  Mode=Multidimensional array
  M : Outport
  wires:
  Matrix Concatenate3/1 -> Matrix Concatenate6/3
  Matrix Concatenate2/1 -> Matrix Concatenate6/2
  Matrix Concatenate1/1 -> Matrix Concatenate6/1
  Demux/3 -> Matrix Concatenate3/1  "a2"
  Demux/5 -> Matrix Concatenate2/2, Matrix Concatenate3/3  "b1"
  Demux/2 -> Matrix Concatenate2/1  "a1"
  " "/1 -> Matrix Concatenate1/3, Matrix Concatenate3/2
  Demux/4 -> Matrix Concatenate1/2, Matrix Concatenate2/3  "b0"
  Demux/1 -> Matrix Concatenate1/1  "a0"
  Matrix Concatenate6/1 -> M/1, Display/1
  In1/1 -> Demux/1

== system rst_auto_reg_Prototipo/RST3/Matrix Q ==
  P1 : Inport
  a1 : Inport  Port=2
  a2 : Inport  Port=3
  R0 : Inport  Port=4
  P2 : Inport  Port=5
  0 : Constant  Value=0
  Display : Display
  Matrix Concatenate : Concatenate  NumInputs=3  Mode=Multidimensional array
  Product : Product
  Product1 : Product
  Sum : Sum  Inputs=-+|
  Sum1 : Sum  Inputs=|+-
  Q : Outport
  wires:
  a2/1 -> Product1/1
  Product1/1 -> Sum1/2
  0/1 -> Matrix Concatenate/3
  Sum1/1 -> Matrix Concatenate/2
  P2/1 -> Sum1/1
  Product/1 -> Sum/1
  R0/1 -> Product/2, Product1/2
  a1/1 -> Product/1
  Sum/1 -> Matrix Concatenate/1
  P1/1 -> Sum/2
  Matrix Concatenate/1 -> Display/1, Q/1

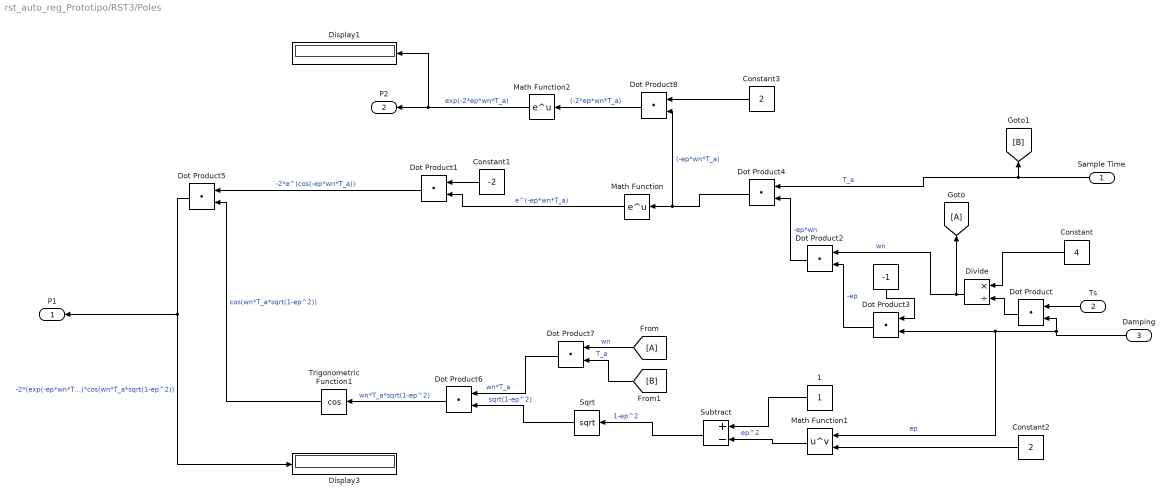
== system rst_auto_reg_Prototipo/RST3/Poles ==
  Sample Time : Inport
  Ts : Inport  Port=2
  Damping : Inport  Port=3
  " " : Constant  Value=-1
  1 : Constant
  Constant : Constant  Value=4
  Constant1 : Constant  Value=-2
  Constant2 : Constant  Value=2
  Constant3 : Constant  Value=2
  Display1 : Display
  Display3 : Display
  Divide : Product  Inputs=*/
  Dot Product{,1..8} (9 alike) : DotProduct  InputSameDT=on  OutDataTypeStr=Inherit: Inherit via internal rule
  Math Function : Math  SaturateOnIntegerOverflow=on
  Math Function1 : Math  Operator=pow  SaturateOnIntegerOverflow=on
  Math Function2 : Math  SaturateOnIntegerOverflow=on
  Sqrt : Sqrt  SaturateOnIntegerOverflow=on
  Subtract : Sum  Inputs=+-
  Trigonometric Function1 : Trigonometry  Operator=cos
  P1 : Outport
  P2 : Outport  Port=2
  wires:
  Math Function2/1 -> P2/1, Display1/1  "exp(-2*ep*wn*T_a)"
  Dot Product8/1 -> Math Function2/1  "(-2*ep*wn*T_a)"
  Constant3/1 -> Dot Product8/1
  Subtract/1 -> Sqrt/1  "1-ep^2"
  Sqrt/1 -> Dot Product6/2  "sqrt(1-ep^2)"
  Dot Product4/1 -> Math Function/1, Dot Product8/2  "(-ep*wn*T_a)"
  Dot Product6/1 -> Trigonometric Function1/1  "wn*T_a*sqrt(1-ep^2)"
  [B] -> Dot Product7/2  "T_a"
  Dot Product2/1 -> Dot Product4/2  "-ep*wn"
  Constant1/1 -> Dot Product1/1
  1/1 -> Subtract/1
  Constant2/1 -> Math Function1/2
  Dot Product1/1 -> Dot Product5/1  "-2*e^(cos(-ep*wn*T_a))"
  Math Function1/1 -> Subtract/2  "ep^2"
  Sample Time/1 -> [B], Dot Product4/1  "T_a"
  Dot Product7/1 -> Dot Product6/1  "wn*T_a"
  Constant/1 -> Divide/1
  Damping/1 -> Dot Product/2, Dot Product3/2, Math Function1/1  "ep"
  Dot Product3/1 -> Dot Product2/2  "-ep"
  Dot Product/1 -> Divide/2
  Ts/1 -> Dot Product/1
  Trigonometric Function1/1 -> Dot Product5/2  "cos(wn*T_a*sqrt(1-ep^2))"
  Dot Product5/1 -> Display3/1, P1/1  "-2*(exp(-ep*wn*T_a))*cos(wn*T_a*sqrt(1-ep^2))"
  " "/1 -> Dot Product3/1
  [A] -> Dot Product7/1  "wn"
  Divide/1 -> Dot Product2/1, [A]  "wn"
  Math Function/1 -> Dot Product1/2  "e^(-ep*wn*T_a)"

== system rst_auto_reg_Prototipo/RST3/Safe division ==
  In1 : Inport
  In2 : Inport  Port=2
  " ESP(0)1" : Constant  Value=eps(0)
  Divide3 : Product  Inputs=*/
  Switch1 : Switch  Criteria=u2 > Threshold
  Out1 : Outport
  wires:
  Switch1/1 -> Divide3/2
  " ESP(0)1"/1 -> Switch1/3
  In2/1 -> Switch1/1, Switch1/2
  In1/1 -> Divide3/1
  Divide3/1 -> Out1/1

== system rst_auto_reg_Prototipo/RST3/Safe division1 ==
  In1 : Inport
  In2 : Inport  Port=2
  " ESP(0)1" : Constant  Value=eps(0)
  Divide3 : Product  Inputs=*/
  Switch1 : Switch  Criteria=u2 > Threshold
  Out1 : Outport
  wires:
  Switch1/1 -> Divide3/2
  " ESP(0)1"/1 -> Switch1/3
  In2/1 -> Switch1/1, Switch1/2
  In1/1 -> Divide3/1
  Divide3/1 -> Out1/1

== system rst_auto_reg_Prototipo/Subsystem1/Subsystem1 ==
  u : Inport
  y : Inport  Port=2
  Delay{,1..5} (6 alike) : Delay  DelayLength=1  InitialCondition=0  SampleTime=0.1
  Mux : Mux  Inputs=3
  Mux1 : Mux  Inputs=3
  Mux2 : Mux  Inputs=2
  re : Outport
  wires:
  Delay4/1 -> Mux1/2, Delay5/1
  u/1 -> Delay/1
  Delay5/1 -> Mux1/3
  Delay/1 -> Mux/1, Delay1/1
  Mux1/1 -> Mux2/2
  Delay1/1 -> Mux/2, Delay2/1
  Mux/1 -> Mux2/1
  Mux2/1 -> re/1
  Delay3/1 -> Mux1/1, Delay4/1
  Delay2/1 -> Mux/3
  y/1 -> Delay3/1

== system rst_auto_reg_Prototipo/Subsystem2/Subsystem1 ==
  u : Inport
  y : Inport  Port=2
  Delay{1..2,4..5} (4 alike) : Delay  DelayLength=1  InitialCondition=0  SampleTime=0.1
  Mux : Mux  Inputs=3
  Mux1 : Mux  Inputs=2
  Mux2 : Mux  Inputs=2
  re : Outport
  wires:
  Delay4/1 -> Mux1/1, Delay5/1
  Mux1/1 -> Mux2/2
  Delay1/1 -> Mux/2, Delay2/1
  Mux/1 -> Mux2/1
  Mux2/1 -> re/1
  u/1 -> Delay4/1
  Delay2/1 -> Mux/3
  y/1 -> Mux/1, Delay1/1
  Delay5/1 -> Mux1/2

== system rst_auto_reg_Prototipo/Subsystem3/Subsystem1 ==
  u : Inport
  y : Inport  Port=2
  Delay{1..2,4..5} (4 alike) : Delay  DelayLength=1  InitialCondition=0  SampleTime=0.1
  Mux : Mux  Inputs=3
  Mux1 : Mux  Inputs=2
  Mux2 : Mux  Inputs=2
  re : Outport
  wires:
  Delay4/1 -> Mux1/1, Delay5/1
  Mux1/1 -> Mux2/2
  Delay1/1 -> Mux/2, Delay2/1
  Mux/1 -> Mux2/1
  Mux2/1 -> re/1
  u/1 -> Delay4/1
  Delay2/1 -> Mux/3
  y/1 -> Mux/1, Delay1/1
  Delay5/1 -> Mux1/2
